simulink model "Energy_consumption_model_V3"  (R2022b)
settings: Solver=VariableStepAuto  StartTime=0.0  StopTime=110  RelTol=1e-3
undefined symbols (not defined in the file or in its folder): arr_db, arr_fg, arr_l, arr_lm, arr_mc1, arr_mc2, arr_mc3, arr_mc4, arr_mc5, arr_rg1, arr_rg2, arr_wc, EC_db, EC_fg, EC_l, EC_lm, EC_mc1, EC_mc2, EC_mc3, EC_mc4, EC_mc5, EC_rg1, EC_rg2, EC_wc, m, msg1, msg2, msg3, msg4, msg5, msgdb, msgfg, msgl, msglm, msgrg1, msgrg2, msgwc, n
(part 2 of 2)

== matlab function Energy_consumption_model_V3/Simulink Function14/MATLAB Function ==
  data: ct_ectm5 input; ECTM5 output
function ECTM5 = fcn(ct_ectm5)
% Define count for counting and prevtime for previous time stamp
persistent pt_ectm5 Ecut_TM5;
% Check if prevtime is empty and initiate the count
if isempty(pt_ectm5)
    pt_ectm5 = ct_ectm5;
    Ecut_TM5 = 0
end
% Increase count by 1 for equal time stamps.
if isequal(ct_ectm5, pt_ectm5)
        Ecut_TM5 = 2000
% Reset count to 1 if two consequitive time stamps are not identical  
elseif Ecut_TM5 ~= 2000
    pt_ectm5 = ct_ectm5;
        Ecut_TM5 = 2000
else
    Ecut_TM5 = 0
end
% Output count for visualization
ECTM5 = Ecut_TM5
end

== matlab function Energy_consumption_model_V3/MATLAB Function4 ==
  data: x input; EB5 output
function EB5 = fcn(x) %x is the time, u1 is 1 = product in pre-cut, u2 = products departed from pre-cut, a is part arrived at pre-cut)
persistent Ebase5 
if isempty(Ebase5)
    Ebase5 = 0
end
if  Ebase5 ~= 500
    Ebase5 = 500
end

EB5 = Ebase5;

== matlab function Energy_consumption_model_V3/Simulink Function/MATLAB Function ==
  data: ct_ertm1 input; ERTM1 output
function ERTM1 = fcn(ct_ertm1)
% Define count for counting and prevtime for previous time stamp
persistent pt_ertm1 EreadyTM1;
ct_ertm1;
% Check if prevtime is empty and initiate the count
if isempty(pt_ertm1)
    pt_ertm1 = ct_ertm1;
    EreadyTM1 = 0;
end
% Increase count by 1 for equal time stamps.
if isequal(ct_ertm1, pt_ertm1)
        EreadyTM1 = 500;
% Reset count to 1 if two consequitive time stamps are not identical  
elseif EreadyTM1 ~= 500
    pt_ertm1 = ct_ertm1;
     EreadyTM1 = 500;
else
    EreadyTM1 = 0;
end
% Output count for visualization
ERTM1 = EreadyTM1;
end

== matlab function Energy_consumption_model_V3/Simulink Function15/MATLAB Function ==
  data: ct_errg1 input; ERRG1 output
function ERRG1 = fcn(ct_errg1)
% Define count for counting and prevtime for previous time stamp
persistent pt_errg1 EreadyRG1;
% Check if prevtime is empty and initiate the count
if isempty(pt_errg1)
    pt_errg1 = ct_errg1;
    EreadyRG1 = 0;
end
% Increase count by 1 for equal time stamps.
if isequal(ct_errg1, pt_errg1)
        EreadyRG1 = 500;
% Reset count to 1 if two consequitive time stamps are not identical  
elseif EreadyRG1 ~= 500
    pt_errg1 = ct_errg1;
        EreadyRG1 = 500;
else
    EreadyRG1 = 0;
end
% Output count for visualization
ERRG1 = EreadyRG1;
end

== matlab function Energy_consumption_model_V3/Simulink Function17/MATLAB Function ==
  data: ct_ecrg1 input; ECRG1 output
function ECRG1 = fcn(ct_ecrg1)
% Define count for counting and prevtime for previous time stamp
persistent pt_ecrg1 Ecut_RG1;
% Check if prevtime is empty and initiate the count
if isempty(pt_ecrg1)
    pt_ecrg1 = ct_ecrg1;
    Ecut_RG1 = 0;
end
% Increase count by 1 for equal time stamps.
if isequal(ct_ecrg1, pt_ecrg1)
        Ecut_RG1 = 2000;
% Reset count to 1 if two consequitive time stamps are not identical  
elseif Ecut_RG1 ~= 2000
    pt_ecrg1 = ct_ecrg1;
        Ecut_RG1 = 2000;
else
    Ecut_RG1 = 0;
end
% Output count for visualization
ECRG1 = Ecut_RG1;
end

== matlab function Energy_consumption_model_V3/MATLAB Function5 ==
  data: x input; EBR1 output
function EBR1 = fcn(x) %x is the time, u1 is 1 = product in pre-cut, u2 = products departed from pre-cut, a is part arrived at pre-cut)
persistent Ebr1 
if isempty(Ebr1)
    Ebr1 = 0;
end
if  Ebr1 ~= 500
    Ebr1 = 500;
end

EBR1 = Ebr1;

== matlab function Energy_consumption_model_V3/Simulink Function18/MATLAB Function ==
  data: ct_errg2 input; ERRG2 output
function ERRG2 = fcn(ct_errg2)
% Define count for counting and prevtime for previous time stamp
persistent pt_errg2 EreadyRG2;
% Check if prevtime is empty and initiate the count
if isempty(pt_errg2)
    pt_errg2 = ct_errg2;
    EreadyRG2 = 0;
end
% Increase count by 1 for equal time stamps.
if isequal(ct_errg2, pt_errg2)
        EreadyRG2 = 500;
% Reset count to 1 if two consequitive time stamps are not identical  
elseif EreadyRG2 ~= 500
    pt_errg2 = ct_errg2;
        EreadyRG2 = 500;
else
    EreadyRG2 = 0;
end
% Output count for visualization
ERRG2 = EreadyRG2;
end

== matlab function Energy_consumption_model_V3/Simulink Function20/MATLAB Function ==
  data: ct_ecrg2 input; ECRG2 output
function ECRG2 = fcn(ct_ecrg2)
% Define count for counting and prevtime for previous time stamp
persistent pt_ecrg2 Ecut_RG2;
% Check if prevtime is empty and initiate the count
if isempty(pt_ecrg2)
    pt_ecrg2 = ct_ecrg2;
    Ecut_RG2 = 0;
end
% Increase count by 1 for equal time stamps.
if isequal(ct_ecrg2, pt_ecrg2)
        Ecut_RG2 = 2000;
% Reset count to 1 if two consequitive time stamps are not identical  
elseif Ecut_RG2 ~= 2000
    pt_ecrg2 = ct_ecrg2;
        Ecut_RG2 = 2000;
else
    Ecut_RG2 = 0;
end
% Output count for visualization
ECRG2 = Ecut_RG2;
end

== matlab function Energy_consumption_model_V3/MATLAB Function6 ==
  data: x input; EBR2 output
function EBR2 = fcn(x) %x is the time, u1 is 1 = product in pre-cut, u2 = products departed from pre-cut, a is part arrived at pre-cut)
persistent Ebr2 
if isempty(Ebr2)
    Ebr2 = 0;
end
if  Ebr2 ~= 500
    Ebr2 = 500;
end

EBR2 = Ebr2;

== matlab function Energy_consumption_model_V3/Simulink Function21/MATLAB Function ==
  data: ct_erlm input; ERLM output
function ERLM = fcn(ct_erlm)
% Define count for counting and prevtime for previous time stamp
persistent pt_erlm Ereadylm;
% Check if prevtime is empty and initiate the count
if isempty(pt_erlm)
    pt_erlm = ct_erlm;
    Ereadylm = 0
end
% Increase count by 1 for equal time stamps.
if isequal(ct_erlm, pt_erlm)
        Ereadylm = 500
% Reset count to 1 if two consequitive time stamps are not identical  
elseif Ereadylm ~= 500
    pt_erlm = ct_erlm;
        Ereadylm = 500
else
    Ereadylm = 0
end
% Output count for visualization
ERLM = Ereadylm
end

== matlab function Energy_consumption_model_V3/Simulink Function23/MATLAB Function ==
  data: ct_eclm input; ECLM output
function ECLM = fcn(ct_eclm)
% Define count for counting and prevtime for previous time stamp
persistent pt_eclm Ecut_lm;
% Check if prevtime is empty and initiate the count
if isempty(pt_eclm)
    pt_eclm = ct_eclm;
    Ecut_lm = 0
end
% Increase count by 1 for equal time stamps.
if isequal(ct_eclm, pt_eclm)
        Ecut_lm = 2000
% Reset count to 1 if two consequitive time stamps are not identical  
elseif Ecut_lm ~= 2000
    pt_eclm = ct_eclm;
        Ecut_lm = 2000
else
    Ecut_lm = 0
end
% Output count for visualization
ECLM = Ecut_lm
end

== matlab function Energy_consumption_model_V3/MATLAB Function7 ==
  data: x input; EBLM output
function EBLM = fcn(x) %x is the time, u1 is 1 = product in pre-cut, u2 = products departed from pre-cut, a is part arrived at pre-cut)
persistent Ebaselm 
if isempty(Ebaselm)
    Ebaselm = 0
end
if  Ebaselm ~= 500
    Ebaselm = 500
end

EBLM = Ebaselm;

== matlab function Energy_consumption_model_V3/Simulink Function24/MATLAB Function ==
  data: ct_erdb input; ERDB output
function ERDB = fcn(ct_erdb)
% Define count for counting and prevtime for previous time stamp
persistent pt_erdb Ereadydb;
% Check if prevtime is empty and initiate the count
if isempty(pt_erdb)
    pt_erdb = ct_erdb;
    Ereadydb = 0
end
% Increase count by 1 for equal time stamps.
if isequal(ct_erdb, pt_erdb)
        Ereadydb = 500
% Reset count to 1 if two consequitive time stamps are not identical  
elseif Ereadydb ~= 500
    pt_erdb = ct_erdb;
        Ereadydb = 500
else
    Ereadydb = 0
end
% Output count for visualization
ERDB = Ereadydb
end

== matlab function Energy_consumption_model_V3/MATLAB Function ==
  data: x input; EB1 output
function EB1 = fcn(x) %x is the time, u1 is 1 = product in pre-cut, u2 = products departed from pre-cut, a is part arrived at pre-cut)
persistent Ebase 
if isempty(Ebase)
    Ebase = 0
end
if Ebase ~= 500
    Ebase = 500
end
EB1 = Ebase;

== matlab function Energy_consumption_model_V3/Simulink Function26/MATLAB Function ==
  data: ct_ecdb input; ECDB output
function ECDB = fcn(ct_ecdb)
% Define count for counting and prevtime for previous time stamp
persistent pt_ecdb Ecut_db;
% Check if prevtime is empty and initiate the count
if isempty(pt_ecdb)
    pt_ecdb = ct_ecdb;
    Ecut_db = 0
end
% Increase count by 1 for equal time stamps.
if isequal(ct_ecdb, pt_ecdb)
        Ecut_db = 2000
% Reset count to 1 if two consequitive time stamps are not identical  
elseif Ecut_db ~= 2000
    pt_ecdb = ct_ecdb;
        Ecut_db = 2000
else
    Ecut_db = 0
end
% Output count for visualization
ECDB = Ecut_db
end

== matlab function Energy_consumption_model_V3/MATLAB Function8 ==
  data: x input; EBDB output
function EBDB = fcn(x) %x is the time, u1 is 1 = product in pre-cut, u2 = products departed from pre-cut, a is part arrived at pre-cut)
persistent Ebasedb 
if isempty(Ebasedb)
    Ebasedb = 0;
end
if  Ebasedb ~= 500
    Ebasedb = 500;
end

EBDB = Ebasedb;

== matlab function Energy_consumption_model_V3/Simulink Function27/MATLAB Function ==
  data: ct_erfg input; ERFG output
function ERFG = fcn(ct_erfg)
% Define count for counting and prevtime for previous time stamp
persistent pt_erfg Ereadyfg;
% Check if prevtime is empty and initiate the count
if isempty(pt_erfg)
    pt_erfg = ct_erfg;
    Ereadyfg = 0
end
% Increase count by 1 for equal time stamps.
if isequal(ct_erfg, pt_erfg)
        Ereadyfg = 500
% Reset count to 1 if two consequitive time stamps are not identical  
elseif Ereadyfg ~= 500
    pt_erfg = ct_erfg;
        Ereadyfg = 500
else
    Ereadyfg = 0
end
% Output count for visualization
ERFG = Ereadyfg
end

== matlab function Energy_consumption_model_V3/Simulink Function29/MATLAB Function ==
  data: ct_ecfg input; ECFG output
function ECFG = fcn(ct_ecfg)
% Define count for counting and prevtime for previous time stamp
persistent pt_ecfg Ecut_fg;
% Check if prevtime is empty and initiate the count
if isempty(pt_ecfg)
    pt_ecfg = ct_ecfg;
    Ecut_fg = 0
end
% Increase count by 1 for equal time stamps.
if isequal(ct_ecfg, pt_ecfg)
        Ecut_fg = 2000
% Reset count to 1 if two consequitive time stamps are not identical  
elseif Ecut_fg ~= 2000
    pt_ecfg = ct_ecfg;
        Ecut_fg = 2000
else
    Ecut_fg = 0
end
% Output count for visualization
ECFG = Ecut_fg
end

== matlab function Energy_consumption_model_V3/MATLAB Function9 ==
  data: x input; EBFG output
function EBFG = fcn(x) %x is the time, u1 is 1 = product in pre-cut, u2 = products departed from pre-cut, a is part arrived at pre-cut)
persistent Ebasefg 
if isempty(Ebasefg)
    Ebasefg = 0
end
if  Ebasefg ~= 500
    Ebasefg = 500
end

EBFG = Ebasefg;

== matlab function Energy_consumption_model_V3/Simulink Function30/MATLAB Function ==
  data: ct_erwc input; ERWC output
function ERWC = fcn(ct_erwc)
% Define count for counting and prevtime for previous time stamp
persistent pt_erwc Ereadywc;
% Check if prevtime is empty and initiate the count
if isempty(pt_erwc)
    pt_erwc = ct_erwc;
    Ereadywc = 0;
end
% Increase count by 1 for equal time stamps.
if isequal(ct_erwc, pt_erwc)
        Ereadywc = 500;
% Reset count to 1 if two consequitive time stamps are not identical  
elseif Ereadywc ~= 500
    pt_erwc = ct_erwc;
        Ereadywc = 500;
else
    Ereadywc = 0;
end
% Output count for visualization
ERWC = Ereadywc;
end

== matlab function Energy_consumption_model_V3/Simulink Function32/MATLAB Function ==
  data: ct_ecwc input; ECWC output
function ECWC = fcn(ct_ecwc)
% Define count for counting and prevtime for previous time stamp
persistent pt_ecwc Ecut_wc;
% Check if prevtime is empty and initiate the count
if isempty(pt_ecwc)
    pt_ecwc = ct_ecwc;
    Ecut_wc = 0;
end
% Increase count by 1 for equal time stamps.
if isequal(ct_ecwc, pt_ecwc)
        Ecut_wc = 2000;
% Reset count to 1 if two consequitive time stamps are not identical  
elseif Ecut_wc ~= 2000
    pt_ecwc = ct_ecwc;
        Ecut_wc = 2000;
else
    Ecut_wc = 0;
end
% Output count for visualization
ECWC = Ecut_wc;
end

== matlab function Energy_consumption_model_V3/MATLAB Function10 ==
  data: x input; EBWC output
function EBWC = fcn(x) %x is the time, u1 is 1 = product in pre-cut, u2 = products departed from pre-cut, a is part arrived at pre-cut)
persistent Ebasewc 
if isempty(Ebasewc)
    Ebasewc = 0
end
if  Ebasewc ~= 500
    Ebasewc = 500
end

EBWC = Ebasewc;

== matlab function Energy_consumption_model_V3/Simulink Function33/MATLAB Function ==
  data: ct_erwc input; ERWC output
function ERWC = fcn(ct_erwc)
% Define count for counting and prevtime for previous time stamp
persistent pt_erwc Ereadywc;
% Check if prevtime is empty and initiate the count
if isempty(pt_erwc)
    pt_erwc = ct_erwc;
    Ereadywc = 0
end
% Increase count by 1 for equal time stamps.
if isequal(ct_erwc, pt_erwc)
        Ereadywc = 500
% Reset count to 1 if two consequitive time stamps are not identical  
elseif Ereadywc ~= 500
    pt_erwc = ct_erwc;
        Ereadywc = 500
else
    Ereadywc = 0
end
% Output count for visualization
ERWC = Ereadywc
end

== matlab function Energy_consumption_model_V3/Simulink Function35/MATLAB Function ==
  data: ct_ecwc input; ECWC output
function ECWC = fcn(ct_ecwc)
% Define count for counting and prevtime for previous time stamp
persistent pt_ecwc Ecut_wc;
% Check if prevtime is empty and initiate the count
if isempty(pt_ecwc)
    pt_ecwc = ct_ecwc;
    Ecut_wc = 0
end
% Increase count by 1 for equal time stamps.
if isequal(ct_ecwc, pt_ecwc)
        Ecut_wc = 2000
% Reset count to 1 if two consequitive time stamps are not identical  
elseif Ecut_wc ~= 2000
    pt_ecwc = ct_ecwc;
        Ecut_wc = 2000
else
    Ecut_wc = 0
end
% Output count for visualization
ECWC = Ecut_wc
end

== matlab function Energy_consumption_model_V3/Simulink Function2/MATLAB Function ==
  data: ct_ectm1 input; ECTM1 output
function ECTM1 = fcn(ct_ectm1)
% Define count for counting and prevtime for previous time stamp
ct_ectm1;
persistent pt_ectm1 Ecut_TM1;
% Check if prevtime is empty and initiate the count
if isempty(pt_ectm1)
    pt_ectm1 = ct_ectm1;
    Ecut_TM1 = 0;
end
% Increase count by 1 for equal time stamps.
if isequal(ct_ectm1, pt_ectm1)
        Ecut_TM1 = 2000;
% Reset count to 1 if two consequitive time stamps are not identical  
elseif Ecut_TM1 ~= 2000
    pt_ectm1 = ct_ectm1;
        Ecut_TM1 = 2000;
else
    Ecut_TM1 = 0;
end
% Output count for visualization
ECTM1 = Ecut_TM1;
end

== matlab function Energy_consumption_model_V3/MATLAB Function11 ==
  data: x input; EBWC output
function EBWC = fcn(x) %x is the time, u1 is 1 = product in pre-cut, u2 = products departed from pre-cut, a is part arrived at pre-cut)
persistent Ebasewc 
if isempty(Ebasewc)
    Ebasewc = 0;
end
if  Ebasewc ~= 500
    Ebasewc = 500;
end

EBWC = Ebasewc;

== matlab function Energy_consumption_model_V3/MATLAB Function12 ==
  data: u input
function fcn(u)
%py_mat_iface(mach_id, mach_stype, mach_energy_used);  
py_mat_iface("1", "turning/milling", u);
end

== matlab function Energy_consumption_model_V3/Simulink Function3/MATLAB Function ==
  data: ct_ertm2 input; ERTM2 output
function ERTM2 = fcn(ct_ertm2)
% Define count for counting and prevtime for previous time stamp
persistent pt_ertm2 EreadyTM2;
% Check if prevtime is empty and initiate the count
if isempty(pt_ertm2)
    pt_ertm2 = ct_ertm2;
    EreadyTM2 = 0;
end
% Increase count by 1 for equal time stamps.
if isequal(ct_ertm2, pt_ertm2)
    EreadyTM2 = 500;
% Reset count to 1 if two consequitive time stamps are not identical  
elseif EreadyTM2 ~= 500
    pt_ertm2 = ct_ertm2;
     EreadyTM2 = 500;
else
    EreadyTM2 = 0;
end
% Output count for visualization
ERTM2 = EreadyTM2;
end

== matlab function Energy_consumption_model_V3/Simulink Function5/MATLAB Function ==
  data: ct_ectm2 input; ECTM2 output
function ECTM2 = fcn(ct_ectm2)
% Define count for counting and prevtime for previous time stamp
persistent pt_ectm2 Ecut_TM2;
% Check if prevtime is empty and initiate the count
if isempty(pt_ectm2)
    pt_ectm2 = ct_ectm2;
    Ecut_TM2 = 0;
end
% Increase count by 1 for equal time stamps.
if isequal(ct_ectm2, pt_ectm2)
        Ecut_TM2 = 2000;
% Reset count to 1 if two consequitive time stamps are not identical  
elseif Ecut_TM2 ~= 2000
    pt_ectm2 = ct_ectm2;
        Ecut_TM2 = 2000;
else
    Ecut_TM2 = 0;
end
% Output count for visualization
ECTM2 = Ecut_TM2;
end

== matlab function Energy_consumption_model_V3/MATLAB Function1 ==
  data: x input; EB2 output
function EB2 = fcn(x) %x is the time, u1 is 1 = product in pre-cut, u2 = products departed from pre-cut, a is part arrived at pre-cut)
persistent Ebase2 
if isempty(Ebase2)
    Ebase2 = 0
end
if  Ebase2 ~= 500
    Ebase2 = 500
end

EB2 = Ebase2;

== matlab function Energy_consumption_model_V3/Simulink Function6/MATLAB Function ==
  data: ct_ertm3 input; ERTM3 output
function ERTM3 = fcn(ct_ertm3)
% Define count for counting and prevtime for previous time stamp
persistent pt_ertm3 EreadyTM3;
% Check if prevtime is empty and initiate the count
if isempty(pt_ertm3)
    pt_ertm3 = ct_ertm3;
    EreadyTM3 = 0;
end
% Increase count by 1 for equal time stamps.
if isequal(ct_ertm3, pt_ertm3)
        EreadyTM3 = 500;
% Reset count to 1 if two consequitive time stamps are not identical  
elseif EreadyTM3 ~= 500
    pt_ertm3 = ct_ertm3;
        EreadyTM3 = 500;
else
    EreadyTM3 = 0;
end
% Output count for visualization
ERTM3 = EreadyTM3;
end

== matlab function Energy_consumption_model_V3/Simulink Function8/MATLAB Function ==
  data: ct_ectm3 input; ECTM3 output
function ECTM3 = fcn(ct_ectm3)
% Define count for counting and prevtime for previous time stamp
persistent pt_ectm3 Ecut_TM3;
% Check if prevtime is empty and initiate the count
if isempty(pt_ectm3)
    pt_ectm3 = ct_ectm3;
    Ecut_TM3 = 0;
end
% Increase count by 1 for equal time stamps.
if isequal(ct_ectm3, pt_ectm3)
        Ecut_TM3 = 2000;
% Reset count to 1 if two consequitive time stamps are not identical  
elseif Ecut_TM3 ~= 2000
    pt_ectm3 = ct_ectm3;
        Ecut_TM3 = 2000;
else
    Ecut_TM3 = 0;
end
% Output count for visualization
ECTM3 = Ecut_TM3;
end

== matlab function Energy_consumption_model_V3/Simulink Function9/MATLAB Function ==
  data: ct_ertm4 input; ERTM4 output
function ERTM4 = fcn(ct_ertm4)
% Define count for counting and prevtime for previous time stamp
persistent pt_ertm4 EreadyTM4;
% Check if prevtime is empty and initiate the count
if isempty(pt_ertm4)
    pt_ertm4 = ct_ertm4;
    EreadyTM4 = 0
end
% Increase count by 1 for equal time stamps.
if isequal(ct_ertm4, pt_ertm4)
        EreadyTM4 = 500
% Reset count to 1 if two consequitive time stamps are not identical  
elseif EreadyTM4 ~= 500
    pt_ertm4 = ct_ertm4;
        EreadyTM4 = 500
else
    EreadyTM4 = 0
end
% Output count for visualization
ERTM4 = EreadyTM4
end

== matlab function Energy_consumption_model_V3/Simulink Function11/MATLAB Function ==
  data: ct_ectm4 input; ECTM4 output
function ECTM4 = fcn(ct_ectm4)
% Define count for counting and prevtime for previous time stamp
persistent pt_ectm4 Ecut_TM4;
% Check if prevtime is empty and initiate the count
if isempty(pt_ectm4)
    pt_ectm4 = ct_ectm4;
    Ecut_TM4 = 0;
end
% Increase count by 1 for equal time stamps.
if isequal(ct_ectm4, pt_ectm4)
        Ecut_TM4 = 2000;
% Reset count to 1 if two consequitive time stamps are not identical  
elseif Ecut_TM4 ~= 2000
    pt_ectm4 = ct_ectm4;
        Ecut_TM4 = 2000;
else
    Ecut_TM4 = 0;
end
% Output count for visualization
ECTM4 = Ecut_TM4;
end

== matlab function Energy_consumption_model_V3/MATLAB Function2 ==
  data: x input; EB3 output
function EB3 = fcn(x) %x is the time, u1 is 1 = product in pre-cut, u2 = products departed from pre-cut, a is part arrived at pre-cut)
persistent Ebase3 
if isempty(Ebase3)
    Ebase3 = 0;
end
if  Ebase3 ~= 500
    Ebase3 = 500;
end

EB3 = Ebase3;

== matlab function Energy_consumption_model_V3/MATLAB Function3 ==
  data: x input; EB4 output
function EB4 = fcn(x) %x is the time, u1 is 1 = product in pre-cut, u2 = products departed from pre-cut, a is part arrived at pre-cut)
persistent Ebase4 
if isempty(Ebase4)
    Ebase4 = 0;
end
if  Ebase4 ~= 500
    Ebase4 = 500;
end

EB4 = Ebase4;

== matlab function Energy_consumption_model_V3/Simulink Function12/MATLAB Function ==
  data: ct_ertm5 input; ERTM5 output
function ERTM5 = fcn(ct_ertm5)
% Define count for counting and prevtime for previous time stamp
persistent pt_ertm5 EreadyTM5;
% Check if prevtime is empty and initiate the count
if isempty(pt_ertm5)
    pt_ertm5 = ct_ertm5;
    EreadyTM5 = 0
end
% Increase count by 1 for equal time stamps.
if isequal(ct_ertm5, pt_ertm5)
        EreadyTM5 = 500
% Reset count to 1 if two consequitive time stamps are not identical  
elseif EreadyTM5 ~= 500
    pt_ertm5 = ct_ertm5;
        EreadyTM5 = 500
else
    EreadyTM5 = 0
end
% Output count for visualization
ERTM5 = EreadyTM5
end
